simulink model "quadcop"  (R2025b)
settings: Solver=ode4  StartTime=0.0  StopTime=300  FixedStep=Ts_inner  RelTol=1e-3
undefined symbols (not defined in the file): quadcop, Ts_gcs
libraries: aerolibutil x4, instrumentseriallib x2, sldrtlib x1
settings Model: DataDictionary=project.sldd  Creator=Nick  LastModifiedBy=Rakete
settings SolverCC: AutoInsertRateTranBlk=on

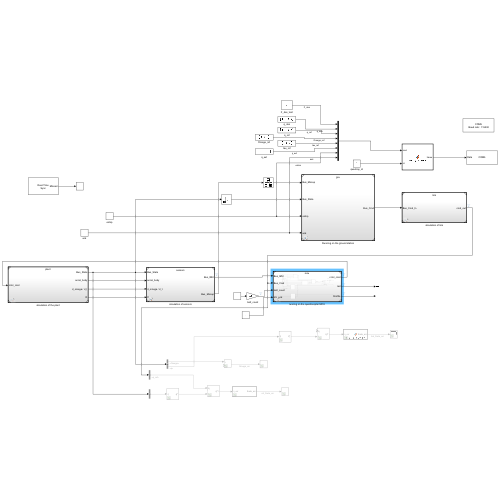
[thumbnail: Simulink's stored preview of the top-level diagram]
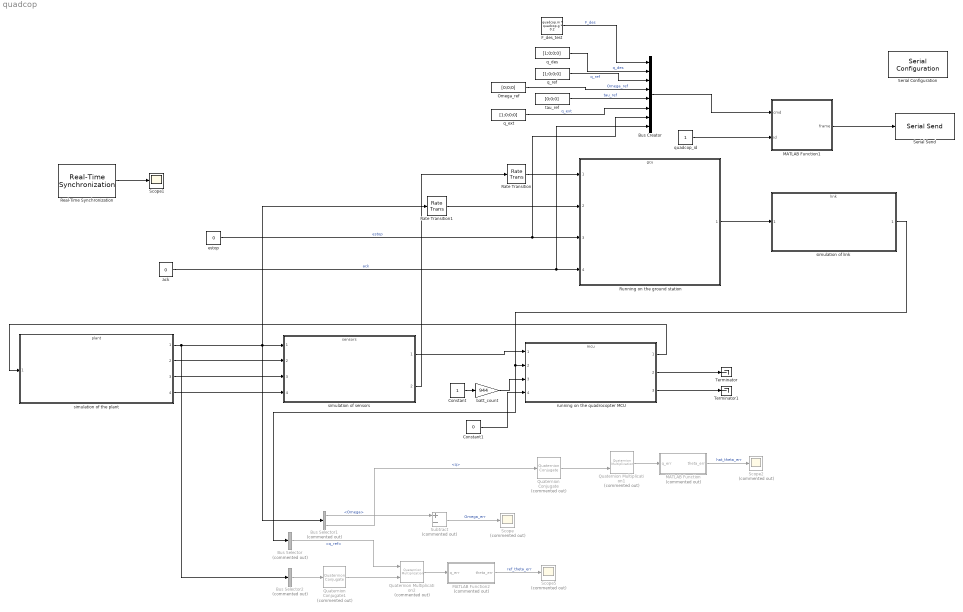
== system quadcop ==
  Bus Creator : BusCreator  Inputs=8  OutDataTypeStr=Bus: Bus_Cmd
  Bus Selector : BusSelector  Commented=on  OutputSignals=q_ref
  Bus Selector1 : BusSelector  Commented=on  OutputSignals=Omega,q
  Bus Selector2 : BusSelector  Commented=on  OutputSignals=q  OutputAsBus=on
  Constant : Constant
  Constant1 : Constant  Value=0  OutDataTypeStr=boolean
  F_des_test : Constant  Value=quadcop.m * quadcop.g * 0.2
  MATLAB Function : MATLAB Function  Commented=on  TreatAsAtomicUnit=on
  MATLAB Function1 : MATLAB Function  TreatAsAtomicUnit=on
  MATLAB Function2 : MATLAB Function  Commented=on  TreatAsAtomicUnit=on
  Omega_ref : Constant  Value=[0;0;0]
  Quaternion Conjugate : aerolibutil/Quaternion Conjugate  Commented=on
  Quaternion Conjugate1 : aerolibutil/Quaternion Conjugate  Commented=on
  Quaternion Multiplication1 : aerolibutil/Quaternion Multiplication  Commented=on
  Quaternion Multiplication2 : aerolibutil/Quaternion Multiplication  Commented=on
  Rate Transition : RateTransition  OutPortSampleTime=Ts_gcs
  Rate Transition1 : RateTransition  OutPortSampleTime=Ts_gcs
  Real-Time Synchronization : sldrtlib/Real-Time Synchronization  SampleTime=Ts_gcs  MaxMissedTicks=inf  ShowMissedTicks=on  YieldWhenWaiting=off
  Running on the ground station : ModelReference  ModelNameDialog=gcu.slx  SimulationMode=Normal  ModelReferenceVersion=1.299
  Scope : Scope  Commented=on
      settings: ActiveDisplayYMinimum=-1  ActiveDisplayYMaximum=1
  Scope1 : Scope
      settings: ActiveDisplayYMinimum=-1  ActiveDisplayYMaximum=1
  Scope2 : Scope  Commented=on
      settings: ActiveDisplayYMinimum=-0.084122920988905683  ActiveDisplayYMaximum=0.78039338720264007  DataLoggingVariableName=ScopeData2
  Scope5 : Scope  Commented=on
      settings: ActiveDisplayYMinimum=-0.013956380673274989  ActiveDisplayYMaximum=0.12560742605947492  DataLoggingVariableName=ScopeData5
  Serial Configuration : instrumentseriallib/Serial Configuration  Priority=-200000  PortSel=COM5  Port=COM5  ComPort=COM5  BaudRate=115200  DataBits=8  Parity=none  StopBits=1  ByteOrder=little-endian  FlowControl=none  Timeout=10  SimulateUsing=Interpreted execution  BlockInModel=on  aMode=1
      settings: LibrarySourceBlock=c2000lib/Host Communication/Serial Configuration
  Serial Send : instrumentseriallib/Serial Send  Priority=1  PortSel=COM5  Port=COM5  ComPort=COM5  Header=[]  Terminator=<none>  CustomTerminator=[]  EnableBlockingMode=on  SimulateUsing=Interpreted execution  BlockInModel=on  aMode=1
      settings: LibrarySourceBlock=c2000lib/Host Communication/Serial Send
  Subtract : Sum  Commented=on  Inputs=+-
  Terminator : Terminator
  Terminator1 : Terminator
  ack : Constant  Value=0  OutDataTypeStr=boolean
  batt_count : Gain  Gain=944
  estop : Constant  Value=0  OutDataTypeStr=uint8
  q_des : Constant  Value=[1;0;0;0]
  q_ext : Constant  Value=[1;0;0;0]
  q_ref : Constant  Value=[1;0;0;0]
  quadcop_id : Constant  OutDataTypeStr=uint8
  running on the quadrocopter MCU : ModelReference  ModelNameDialog=mcu.slx  SimulationMode=Normal  ModelReferenceVersion=1.284
  simulation of link : ModelReference  ModelNameDialog=link.slx  SimulationMode=Normal  ModelReferenceVersion=1.134
  simulation of sensors : ModelReference  ModelNameDialog=sensors.slx  SimulationMode=Normal  ModelReferenceVersion=1.86
  simulation of the plant : ModelReference  ModelNameDialog=plant.slx  SimulationMode=Normal  ModelReferenceVersion=1.208
  tau_ref : Constant  Value=[0;0;0]
  wires:
  simulation of the plant/1 -> Bus Selector2/1, Rate Transition1/1, Bus Selector1/1, simulation of sensors/1
  simulation of the plant/2 -> simulation of sensors/2
  simulation of the plant/3 -> simulation of sensors/3
  simulation of the plant/4 -> simulation of sensors/4
  simulation of sensors/1 -> running on the quadrocopter MCU/1
  simulation of sensors/2 -> Rate Transition/1
  Quaternion Conjugate/1 -> Quaternion Multiplication1/2
  MATLAB Function/1(theta_err) -> Scope2/1  "hat_theta_err"
  Quaternion Multiplication1/1 -> MATLAB Function/1(q_err)
  Bus Selector1/1 -> Subtract/1  "<Omega>"
  Subtract/1 -> Scope/1  "Omega_err"
  Bus Selector1/2 -> Quaternion Conjugate/1  "<q>"
  Bus Selector2/1 -> Quaternion Conjugate1/1
  Quaternion Multiplication2/1 -> MATLAB Function2/1(q_err)
  MATLAB Function2/1(theta_err) -> Scope5/1  "ref_theta_err"
  Quaternion Conjugate1/1 -> Quaternion Multiplication2/2
  Running on the ground station/1 -> simulation of link/1
  Rate Transition/1 -> Running on the ground station/1
  Rate Transition1/1 -> Running on the ground station/2
  Bus Selector/1 -> Quaternion Multiplication2/1  "<q_ref>"
  simulation of link/1 -> Bus Selector/1, running on the quadrocopter MCU/2
  Real-Time Synchronization/1 -> Scope1/1
  estop/1 -> Bus Creator/7, Running on the ground station/3  "estop"
  ack/1 -> Bus Creator/8, Running on the ground station/4  "ack"
  Constant/1 -> batt_count/1
  batt_count/1 -> running on the quadrocopter MCU/3
  running on the quadrocopter MCU/1 -> simulation of the plant/1
  running on the quadrocopter MCU/2 -> Terminator/1
  running on the quadrocopter MCU/3 -> Terminator1/1
  quadcop_id/1 -> MATLAB Function1/2(id)
  MATLAB Function1/1(frame) -> Serial Send/1
  Constant1/1 -> running on the quadrocopter MCU/4
  F_des_test/1 -> Bus Creator/1  "F_des"
  q_des/1 -> Bus Creator/2  "q_des"
  q_ref/1 -> Bus Creator/3  "q_ref"
  Omega_ref/1 -> Bus Creator/4  "Omega_ref"
  tau_ref/1 -> Bus Creator/5  "tau_ref"
  q_ext/1 -> Bus Creator/6  "q_ext"
  Bus Creator/1 -> MATLAB Function1/1(cmd)

== matlab function quadcop/MATLAB Function ==
  data: q_err input; theta_err output
function theta_err = quat_2_rotAngle(q_err)   
%#codegen
    theta_err = 2*atan2(norm(q_err(2:4)), abs(q_err(1)));
end

== matlab function quadcop/MATLAB Function2 ==
  data: q_err input; theta_err output
function theta_err = quat_2_rotAngle(q_err)   %#codegen
    theta_err = 2*atan2(norm(q_err(2:4)), abs(q_err(1)));
end

== matlab function quadcop/MATLAB Function1 ==
  data: cmd input Bus: Bus_Cmd; frame output uint8 size=[1 82]; id input uint8 size=[1 1]
function frame = pack_gcs_frame_sl(cmd, id)
%#codegen
% WRAPPER — haelt KEINE Logik. Single Source of Truth ist
% scripts\functions\pack_gcs_frame.m; dieser Block ruft sie nur auf.
% Grund: .slx ist binaer -> Inline-Kopien driften unbemerkt und sind im
% git-Diff unsichtbar (Session 9: 2 von 11 Bloecken waren abgewichen).
% Name MUSS abweichen (_sl), sonst schattet er die externe Funktion.
frame = pack_gcs_frame(cmd, id);
end
